simulink model "effort_interface"  (R2019b)
settings: Solver=VariableStepAuto  StartTime=0.0  StopTime=10.0  RelTol=1e-3
undefined symbols (not defined in the file or in its folder): Kd, Ki, Kp
settings Model: Creator=AL30832  LastModifiedBy=AL30832

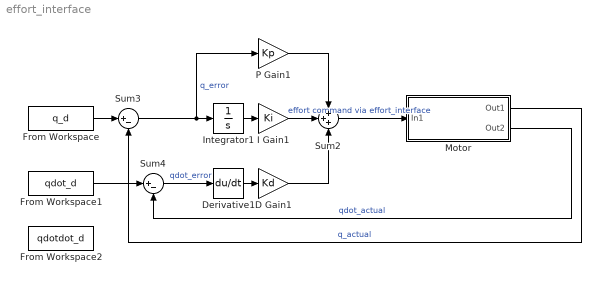
== system effort_interface ==
  D Gain1 : Gain  Gain=Kd
  Derivative1 : Derivative  CoefficientInTFapproximation=Derivative
  From Workspace : FromWorkspace  VariableName=q_d  SampleTime=0
  From Workspace1 : FromWorkspace  VariableName=qdot_d  SampleTime=0
  From Workspace2 : FromWorkspace  VariableName=qdotdot_d  SampleTime=0
  I Gain1 : Gain  Gain=Ki
  Integrator1 : Integrator
  Motor : Subsystem
  P Gain1 : Gain  Gain=Kp
  Sum2 : Sum  Inputs=+++
  Sum3 : Sum  Inputs=|+-
  Sum4 : Sum  Inputs=|+-
  wires:
  Derivative1/1 -> D Gain1/1
  D Gain1/1 -> Sum2/3
  Sum3/1 -> Integrator1/1, P Gain1/1  "q_error"
  From Workspace1/1 -> Sum4/1
  Motor/1(Out1) -> Sum3/2  "q_actual"
  Sum4/1 -> Derivative1/1  "qdot_error"
  Motor/2(Out2) -> Sum4/2  "qdot_actual"
  Sum2/1 -> Motor/1(In1)  "effort command via effort_interface"
  P Gain1/1 -> Sum2/1
  I Gain1/1 -> Sum2/2
  Integrator1/1 -> I Gain1/1
  From Workspace/1 -> Sum3/1

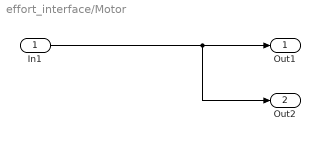
== system effort_interface/Motor ==
  In1 : Inport
  Out1 : Outport
  Out2 : Outport  Port=2
  wires:
  In1/1 -> Out2/1, Out1/1
